simulink model "CompLab1_1"  (R2020a)
settings: Solver=VariableStepAuto  StartTime=0.0  StopTime=20.0  RelTol=1e-3
undefined symbols (not defined in the file): stepf, stepi, stept, tau, x0
settings Model: Creator=cal  LastModifiedBy=cal
settings DataIOCC: ReturnWorkspaceOutputs=off  TimeSaveName=mytime  OutputSaveName=x

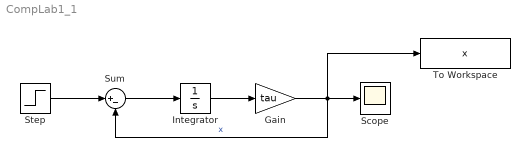
== system CompLab1_1 ==
  Gain : Gain  Gain=tau
  Integrator : Integrator  InitialCondition=x0
  Scope : Scope
  Step : Step  Time=stept  Before=stepi  After=stepf  SampleTime=0
  Sum : Sum  Inputs=|+-
  To Workspace : ToWorkspace  VariableName=x  SampleTime=-1
  wires:
  Step/1 -> Sum/1
  Sum/1 -> Integrator/1
  Integrator/1 -> Gain/1
  Gain/1 -> To Workspace/1, Sum/2, Scope/1  "x"
